simulink model "B2B_HVDC_MMC"  (R2023b)
settings: Solver=ode23t  StartTime=0.0  StopTime=3  FixedStep=Ts_Power  MaxStep=1e-3  MinStep=Ts_Power  RelTol=1e-3
values from neighbouring files (symbols this model uses):
  AC_lim = 1*[1.5 -1.5]    [B2B_HVDC_MMC_Calc.m]
  C_pm = 10.48e-3    (= 0.01048)    [B2B_HVDC_MMC_Calc.m]
  Carm = 1.0*C_pm/n    (= 0.0002096)    [B2B_HVDC_MMC_Calc.m]    (also in HVDC_MMC_param.m = 4.88333333333e-05)
  ccsc_lim = 1*[1.0 -1.0]    [B2B_HVDC_MMC_Calc.m]
  DC_lim = 1*[1.05 -1.05]    [B2B_HVDC_MMC_Calc.m]
  f = 50    [B2B_HVDC_MMC_Calc.m]
  Fn_filter = 1000    [B2B_HVDC_MMC_Calc.m]    (also in HVDC_MMC_param.m)
  Fnom = 50    [HVDC_MMC_param.m]
  HrmOrd = N    (= 2)    [B2B_HVDC_MMC_Calc.m]    (also in HVDC_MMC_param.m)
  I_nom = S_nom/(sqrt(3)*V_grid)    [B2B_HVDC_MMC_Calc.m]
  Ireg_lim_i = 1*[1.5, -1.5]    [B2B_HVDC_MMC_Calc.m]
  Ireg_lim_r = 2*[1.5, -1.5]    [B2B_HVDC_MMC_Calc.m]
  Ki_ACreg_i = 260    [B2B_HVDC_MMC_Calc.m]
  Ki_ccsc = 5    [B2B_HVDC_MMC_Calc.m]
  Ki_DCreg_r = 150    [B2B_HVDC_MMC_Calc.m]
  Ki_Ireg_i = 200    [B2B_HVDC_MMC_Calc.m]
  Ki_Ireg_r = 50    [B2B_HVDC_MMC_Calc.m]
  Kp_ACreg_i = 2    [B2B_HVDC_MMC_Calc.m]
  Kp_ccsc = 1    [B2B_HVDC_MMC_Calc.m]
  Kp_DCreg_r = 8    [B2B_HVDC_MMC_Calc.m]
  Kp_Ireg_i = 2    [B2B_HVDC_MMC_Calc.m]
  Kp_Ireg_r = 0.8    [B2B_HVDC_MMC_Calc.m]
  L1_si = L1_pu*Z_base66/w    [B2B_HVDC_MMC_Calc.m]
  L_arm = L_arm_pu*Z_base66/w    [B2B_HVDC_MMC_Calc.m]
  L_arm_pu = 0.15    [B2B_HVDC_MMC_Calc.m]
  N = 2    [B2B_HVDC_MMC_Calc.m]
  P_nom = 220e6    (= 220000000)    [B2B_HVDC_MMC_Calc.m]
  R1_si = R1_pu*Z_base66    [B2B_HVDC_MMC_Calc.m]
  R_arm = 0.03    [B2B_HVDC_MMC_Calc.m]
  R_arm_pu = R_arm/Z_base66    [B2B_HVDC_MMC_Calc.m]
  R_load = 0.6*40    (= 24)    [B2B_HVDC_MMC_Calc.m]
  R_startup = 17    [B2B_HVDC_MMC_Calc.m]    (also in HVDC_MMC_param.m = 400)
  T_fault = 1.4    [B2B_HVDC_MMC_Calc.m]
  Ts = Ts_Power    (= 5e-05)    [B2B_HVDC_MMC_Calc.m]    (also in HVDC_MMC_param.m)
  Ts_Control = Ts_Power    (= 5e-05)    [B2B_HVDC_MMC_Calc.m]    (also in HVDC_MMC_param.m)
  Ts_DQN = MultTs*Ts_Power    (= 5e-05)    [B2B_HVDC_MMC_Calc.m]    (also in HVDC_MMC_param.m)
  Ts_Power = 1*50e-6    (= 5e-05)    [B2B_HVDC_MMC_Calc.m]    (also in HVDC_MMC_param.m)
  V_ac_ref = 1.035    [B2B_HVDC_MMC_Calc.m]
  V_grid = 66e3    (= 66000)    [B2B_HVDC_MMC_Calc.m]
  Vdc_nom = 135e3    (= 135000)    [B2B_HVDC_MMC_Calc.m]
  Vnom_prim = 333e3    (= 333000)    [HVDC_MMC_param.m]
  Xdcpnz = [zeros(6,1), Xpnz]    [B2B_HVDC_MMC_Calc.m]
  Zeta_filter = 1    [B2B_HVDC_MMC_Calc.m]    (also in HVDC_MMC_param.m)
undefined symbols (not defined in the file or in its folder): DiscIntNeverNeededParam, Pcc, Xdcpnz_c
libraries: DQN_Lib x39, simulink x26, eeTransforms x21, spsCurrentMeasurementLib x16, spsHalfBridgeMMCLib x12, spsSeriesRLCBranchLib x12, B2B_HVDC_MMC_Lib x8, spsSecondOrderFilterLib x8, spsAlphaBetaZerotodq0Lib x6, spsabctoAlphaBetaZeroLib x6, spsThreePhaseVIMeasurementLib x4, spsabctodq0Lib x3
(part 3 of 5)

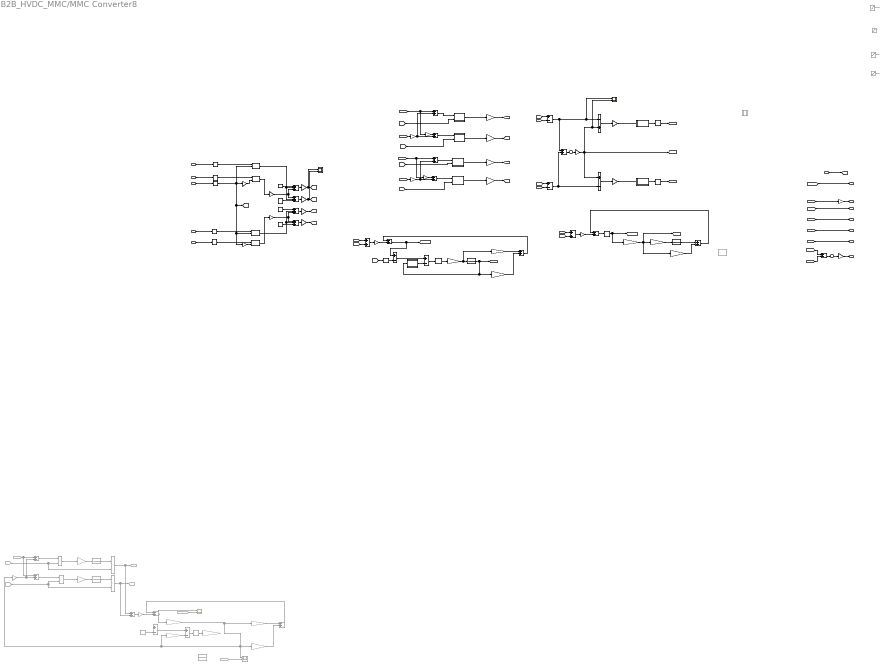
== system B2B_HVDC_MMC/MMC Converter8 ==
  m_dq1_r : Inport
  m_dq2_r : Inport  Port=2
  Vg : Inport  Port=3
  wt : Inport  Port=4
  m_dq1_i : Inport  Port=5
  m_dq2_i : Inport  Port=6
  Add1 : Sum  Inputs=+-
  Add{3,6,38..39,41,44,48,50,73} (9 alike) : Sum
  Add35 : Sum  Commented=on
  Add36 : Sum  Commented=on
  Add37 : Sum  Commented=on  Inputs=-+
  Add4 : Sum  Commented=on
  Add42 : Sum  Inputs=-+
  Add45 : Sum  Inputs=-+
  Add46 : Sum  Inputs=+-
  Add47 : Sum  Inputs=+-
  Add5 : Sum  Commented=on  Inputs=-+
  Constant : Constant  Commented=on  Value=0
  Constant{1..2,74..75} (4 alike) : Constant
  Delay{2..3,8..9} (4 alike) : Delay  DelayLength=1  SampleTime=Ts_Power
  Delay4 : Delay  Commented=on  DelayLength=1  SampleTime=Ts_Power
  Discrete Derivative : simulink/Discrete/Discrete Derivative  Commented=on  gainval=Ts_Power  ICPrevScaledInput=0.0  OutMin=[]  OutMax=[]  OutDataType=fixdt(1, 16)  OutScaling=2^-10  DoSatur=off
  Discrete-Time Integrator : DiscreteIntegrator  IntegratorMethod=Integration: Trapezoidal  SampleTime=Ts_Power  ICPrevOutput=DiscIntNeverNeededParam  ICPrevScaledInput=DiscIntNeverNeededParam
  Discrete-Time Integrator4 : DiscreteIntegrator  Commented=on  IntegratorMethod=Integration: Trapezoidal  SampleTime=Ts_Power  ICPrevOutput=DiscIntNeverNeededParam  ICPrevScaledInput=DiscIntNeverNeededParam
  Discrete-Time Integrator5 : DiscreteIntegrator  Commented=on  IntegratorMethod=Integration: Trapezoidal  SampleTime=Ts_Power  ICPrevOutput=DiscIntNeverNeededParam  ICPrevScaledInput=DiscIntNeverNeededParam
  Discrete-Time Integrator7 : DiscreteIntegrator  IntegratorMethod=Integration: Trapezoidal  SampleTime=Ts_Power  ICPrevOutput=DiscIntNeverNeededParam  ICPrevScaledInput=DiscIntNeverNeededParam
  Discrete-Time Integrator8 : DiscreteIntegrator  Commented=on  IntegratorMethod=Integration: Trapezoidal  SampleTime=Ts_Power  ICPrevOutput=DiscIntNeverNeededParam  ICPrevScaledInput=DiscIntNeverNeededParam
  From108 : From  Commented=on  GotoTag=Id_abc_i
  From51 : From  Commented=on  GotoTag=mn_i
  From56 : From  Commented=on  GotoTag=mp_i
  From72 : From  Commented=on  GotoTag=Ig_abc_i
  From75 : From  Commented=on  GotoTag=Vconv_i
  Gain{1..2,18,23..24} (5 alike) : Gain  Gain=-1
  Gain10 : Gain  Gain=1/6
  Gain12 : Gain  Gain=-2
  Gain13 : Gain  Commented=on  Gain=1/(Carm)
  Gain14 : Gain  Commented=on  Gain=1/(Carm)
  Gain15 : Gain  Commented=on  Gain=0.5
  Gain{3..6} (4 alike) : Gain  Gain=1/(Carm)
  Gain40 : Gain  Commented=on  Gain=-0.5
  Gain41 : Gain  Gain=1/2
  Gain44 : Gain  Gain=0.5
  Gain46 : Gain  Commented=on  Gain=1/R_load
  Gain47 : Gain  Gain=0.5
  Gain49 : Gain  Gain=-0.5
  Gain50 : Gain  Gain=1/R_load
  Gain51 : Gain  Gain=R_arm/2
  Gain52 : Gain  Commented=on  Gain=R_arm/2
  Gain53 : Gain  Commented=on  Gain=L_arm/2
  Gain54 : Gain  Commented=on  Gain=1/L1_si
  Gain55 : Gain  Commented=on  Gain=R1_si+R_load
  Gain56 : Gain  Gain=L_arm/2
  Gain60 : Gain  Gain=-0.5
  Gain61 : Gain  Gain=R_arm/2
  Gain62 : Gain  Gain=L_arm/2
  Gain65 : Gain  Gain=1/L1_si
  Gain9 : Gain  Gain=-2
  Goto56 : Goto  Commented=on  GotoTag=Vp_ic
  Goto57 : Goto  Commented=on  GotoTag=Vn_ic
  I->pu{1..3,5,22,28} (6 alike) : Gain  Gain=1/2  SaturateOnIntegerOverflow=on  OutDataTypeStr=Inherit: Same as input  ParamDataTypeStr=Inherit: Same as input
  Int : MATLAB Function  TreatAsAtomicUnit=on  mask{dt=Ts_Power}
      mask prompts: dt "Time step (s):"
  Int2 : MATLAB Function  TreatAsAtomicUnit=on  mask{dt=Ts_Power}
      mask prompts: dt "Time step (s):"
  Inverse Park Transform{1..4} (4 alike) : eeTransforms/Inverse Park Transform  AxisAlignment=Q-axis  PowerInvariant=off
  MATLAB Function1 : MATLAB Function  TreatAsAtomicUnit=on  mask{dt=Ts_Power}
      mask prompts: dt "Time step (s):"
  MATLAB Function2 : MATLAB Function  TreatAsAtomicUnit=on  mask{dt=Ts_Power}
      mask prompts: dt "Time step (s):"
  MATLAB Function3 : MATLAB Function  TreatAsAtomicUnit=on  mask{dt=Ts_Power}
      mask prompts: dt "Time step (s):"
  MATLAB Function4 : MATLAB Function  TreatAsAtomicUnit=on  mask{dt=Ts_Power}
      mask prompts: dt "Time step (s):"
  Product{1..3,5} (4 alike) : Product  Commented=on
  R_rec1 : Subsystem
  Rate Transition{1..4,10..11} (6 alike) : RateTransition  Integrity=off  OutPortSampleTimeMultiple=MultTs  OutPortSampleTime=Ts_Power
  Saturation3 : Saturate  Commented=on  UpperLimit=inf  LowerLimit=0  ZeroCross=off
  Saturation4 : Saturate  Commented=on  UpperLimit=inf  LowerLimit=0  ZeroCross=off
  Saturation5 : Saturate  Commented=on  UpperLimit=0  LowerLimit=-inf  ZeroCross=off
  Saturation6 : Saturate  Commented=on  UpperLimit=0  LowerLimit=-inf  ZeroCross=off
  Scope : Scope  NumInputPorts=2
  Scope1 : Scope  NumInputPorts=2
  Scope15 : Scope  Commented=on  NumInputPorts=2
  Scope8 : Scope  Commented=on  NumInputPorts=2
  Subsystem2 : Subsystem  Commented=on  mask{Ts_Power=Ts_Power, SW=off}
      mask prompts: Ts_Power "Sample time (s):"; SW "Fancy delay"
  Subtract1 : Sum  Inputs=+-+
  Subtract10 : Sum  Inputs=+-
  Subtract11 : Sum  Inputs=+-
  Subtract2 : Sum  Inputs=+-+
  Subtract3 : Sum  Inputs=+++
  Subtract4 : Sum  Commented=on  Inputs=+-
  Subtract5 : Sum  Inputs=+++
  Subtract8 : Sum  Commented=on  Inputs=+-
  Sum11 : Sum  Inputs=+-  InputSameDT=on  SaturateOnIntegerOverflow=on  OutDataTypeStr=Inherit: Same as first input
  Sum19 : Sum  Inputs=+
  Sum23 : Sum  Inputs=+
  Sum4 : Sum  Inputs=-+  InputSameDT=on  SaturateOnIntegerOverflow=on  OutDataTypeStr=Inherit: Same as first input
  Id_abc_i : Outport  VectorParamsAs1DForOutWhenUnconnected=off
  Ig_abc_i : Outport  Port=2  VectorParamsAs1DForOutWhenUnconnected=off
  Vg_abc_i : Outport  Port=3  VectorParamsAs1DForOutWhenUnconnected=off
  Idc : Outport  Port=4  VectorParamsAs1DForOutWhenUnconnected=off
  Ig_abc_r : Outport  Port=5  VectorParamsAs1DForOutWhenUnconnected=off
  Id_abc_r : Outport  Port=6  VectorParamsAs1DForOutWhenUnconnected=off
  Vdc : Outport  Port=7  VectorParamsAs1DForOutWhenUnconnected=off
  wires:
  Gain9/1 -> Inverse Park Transform2/2
  [mn_r] -> MATLAB Function1/2(y)
  Add6/1 -> MATLAB Function1/1(x)
  Add46/1 -> Scope1/1, Sum4/1, Add73/1  "dVp_M"
  Subtract2/1 -> I->pu22/1
  Constant74/1 -> Subtract2/1
  Inverse Park Transform2/1 -> Gain1/1
  Constant75/1 -> Subtract5/3
  Subtract5/1 -> I->pu28/1
  I->pu28/1 -> Scope/2, [mn_r]
  Inverse Park Transform1/1 -> Subtract5/2, Subtract2/2
  Gain12/1 -> Inverse Park Transform4/2
  wt/1 -> Rate Transition1/1
  Constant2/1 -> Subtract3/3
  Subtract1/1 -> I->pu2/1
  Constant1/1 -> Subtract1/1
  Subtract3/1 -> I->pu3/1
  I->pu2/1 -> [mp_i]
  Inverse Park Transform4/1 -> Gain2/1
  I->pu3/1 -> [mn_i]
  Gain15/1 -> Add4/2, Add5/2
  Discrete-Time Integrator5/1 -> Product2/1  "Vp_M"
  Add5/1 -> Product3/1
  Add4/1 -> Product1/1  "prod"
  Gain14/1 -> Discrete-Time Integrator5/1  "dVp_M"
  Product1/1 -> Gain14/1
  Discrete-Time Integrator4/1 -> Product5/1  "Vn_M"
  Gain13/1 -> Discrete-Time Integrator4/1  "dVn_M"
  Product3/1 -> Gain13/1
  From51/1 -> Product2/2, Product1/2
  From56/1 -> Product3/2, Product5/2
  Vg/1 -> [Vg_r]
  Sum4/1 -> I->pu5/1
  Gain23/1 -> Ig_abc_r/1
  Gain44/1 -> Add6/2, Add3/2
  From75/1 -> Scope8/2
  Constant/1 -> Subtract4/2
  Delay4/1 -> Gain54/1
  Gain55/1 -> Subtract8/2
  Subtract8/1 -> Delay4/1
  Gain53/1 -> Add36/1  "dVp_M"
  Gain52/1 -> Add36/2  "dVp_M"
  Add37/1 -> Scope8/1, Gain46/1  "prod"
  Subtract4/1 -> Subtract8/1
  Product2/1 -> Add35/1, Goto56/1
  Gain46/1 -> Scope15/1, Gain55/1, Gain15/1, Gain52/1, Gain53/1  "Igd"
  Product5/1 -> Add35/2, Goto57/1
  From72/1 -> Scope15/2
  Add36/1 -> Add37/1  "prod"
  Add35/1 -> Gain40/1
  Gain40/1 -> Add37/2  "Vce_i"
  From108/1 -> Add5/1, Add4/1
  Gain47/1 -> Add38/2, Add39/2
  [mp_i] -> MATLAB Function4/2(y)
  Add38/1 -> MATLAB Function3/1(x)  "prod"
  Add39/1 -> MATLAB Function4/1(x)
  [mn_i] -> MATLAB Function3/2(y)
  Add41/1 -> Add42/1  "prod"
  Gain51/1 -> Add41/2  "dVp_M"
  Add50/1 -> Gain49/1
  Gain49/1 -> Add42/2  "Vce_i"
  Subtract10/1 -> Subtract11/1
  Gain61/1 -> Add44/2  "dVp_M"
  Add44/1 -> Add45/1  "prod"
  Gain60/1 -> Add45/2  "Vce_r"
  Gain62/1 -> Add44/1  "dVp_M"
  R_rec1/1(Out) -> Subtract11/2
  Gain65/1 -> Discrete-Time Integrator/1, Gain62/1
  Add48/1 -> Gain60/1
  [Ig_abc_ic] -> Gain47/1
  [Id_abc_ic] -> Gain24/1, Add38/1
  [Vp_rc] -> Add46/1
  [Vn_rc] -> Add46/2
  [Vp_ic] -> Add47/1
  [Vn_ic] -> Add47/2
  [Ig_abc_rc] -> Gain44/1
  [Id_abc_rc] -> Add3/1, Gain18/1
  [Vp_rc] -> Add48/1
  [Vn_rc] -> Add48/2
  [Vp_ic] -> Add50/1
  [Vn_ic] -> Add50/2
  Add47/1 -> Sum11/2, Add73/2  "dVp_M"
  [Ig_abc_rc] -> Gain23/1
  [Id_abc_rc] -> Id_abc_r/1
  [Ig_abc_ic] -> Ig_abc_i/1
  [Id_abc_ic] -> Id_abc_i/1
  [Id_abc_rc] -> Add1/2
  Gain56/1 -> Discrete-Time Integrator7/1  "dVp_M"
  Discrete-Time Integrator7/1 -> Add41/1
  [Id_abc_ic] -> Add1/1
  Add1/1 -> Sum23/1
  Gain41/1 -> Idc/1  "Vce_r"
  Discrete-Time Integrator/1 -> [Ig_abc_rc], R_rec1/1(In), Gain61/1  "Igd"
  Add45/1 -> [Vconv_rc], Subtract10/1  "prod"
  Gain50/1 -> Gain51/1, [Ig_abc_ic], Gain56/1  "Igd"
  Add42/1 -> Delay8/1  "prod"
  [Vconv_ic] -> Vg_abc_i/1
  [V_dc_c] -> Vdc/1
  Subtract11/1 -> Delay9/1
  Gain1/1 -> Subtract5/1, Subtract2/3
  Inverse Park Transform3/1 -> Subtract1/2, Subtract3/2
  Gain2/1 -> Subtract3/1, Subtract1/3
  Gain10/1 -> Sum11/1, Scope1/2, Sum4/2, [V_dc_c]  "Vce_r"
  m_dq2_r/1 -> Rate Transition11/1
  m_dq1_r/1 -> Rate Transition10/1
  m_dq1_i/1 -> Rate Transition2/1
  m_dq2_i/1 -> Rate Transition3/1
  Gain18/1 -> Add6/1
  Gain24/1 -> Add39/1
  Saturation4/1 -> ?
  Saturation3/1 -> ?
  Saturation6/1 -> ?
  Add73/1 -> Sum19/1
  Sum19/1 -> Gain10/1
  Int/1(z) -> Delay2/1
  Sum11/1 -> I->pu1/1
  Int2/1(z) -> Delay3/1
  MATLAB Function3/1(z) -> Gain5/1
  MATLAB Function4/1(z) -> Gain6/1
  Delay2/1 -> [Id_abc_rc]
  Delay3/1 -> [Id_abc_ic]
  Delay9/1 -> Gain65/1
  Delay8/1 -> Gain50/1, [Vconv_ic]
  I->pu5/1 -> Int/1(x)
  I->pu1/1 -> Int2/1(x)
  Rate Transition10/1 -> Inverse Park Transform1/1
  Rate Transition11/1 -> Inverse Park Transform2/1
  Rate Transition1/1 -> [wt], Inverse Park Transform3/2, Gain12/1, Inverse Park Transform1/2, Gain9/1
  Rate Transition2/1 -> Inverse Park Transform3/1
  Rate Transition3/1 -> Inverse Park Transform4/1
  [Vg_r] -> Rate Transition4/1
  Rate Transition4/1 -> Subtract10/2
  Sum23/1 -> Gain41/1
  I->pu22/1 -> Scope/1, [mp_r]
  Add3/1 -> MATLAB Function2/1(x)  "prod"
  [mp_r] -> MATLAB Function2/2(y)
  MATLAB Function2/1(z) -> Gain3/1  "dVp_M"
  Gain3/1 -> [Vp_rc]  "dVp_M"
  MATLAB Function1/1(z) -> Gain4/1  "dVp_M"
  Gain4/1 -> [Vn_rc]  "dVp_M"
  Gain5/1 -> [Vp_ic]  "dVp_M"
  Gain6/1 -> [Vn_ic]  "dVp_M"

== system B2B_HVDC_MMC/Dq0 Control11/Subsystem1 ==
  V_dc_meas : Inport
  Ig_dq1+ : Inport  Port=2
  Vg_dq1+ : Inport  Port=3
  Id_dq2- : Inport  Port=4
  AC Voltage Controller : Subsystem
  Circulating current suppression : Subsystem  VariantControl=Variant1
  Constant1 : Constant  Value=1/(Vdc_nom/2*sqrt(3)/sqrt(2)/V_grid)
  Constant2 : Constant  Value=Vdc_nom
  Constant6 : Constant  Value=V_grid
  DC voltage control - Outer loop : Subsystem
  Gain5 : Gain  Gain=(V_grid)
  Inncer current loop - Positive and Negative Sequence Control : Subsystem
  Interpreted MATLAB Function : MATLABFcn  MATLABFcn=sqrt(u(1)^2+u(2)^2)
  Step : Step  Time=(T_fault+0.15)  Before=[DC_lim(1) DC_lim(2)]  After=[DC_lim(1) DC_lim(2)]  SampleTime=0
  m_dq1 : Outport
  m_dq2 : Outport  Port=2
  wires:
  Interpreted MATLAB Function/1 -> AC Voltage Controller/3(V_ac)
  Vg_dq1+/1 -> Gain5/1, Inncer current loop - Positive and Negative Sequence Control/4(Vdq+)
  [T_circ_r] -> Circulating current suppression/Enable
  [T_iq_reg_r] -> AC Voltage Controller/Enable, AC Voltage Controller/1("Enable ")
  Constant2/1 -> DC voltage control - Outer loop/2(V_dc_ref)
  AC Voltage Controller/1(Iq_ref) -> Inncer current loop - Positive and Negative Sequence Control/2(iq_pos_ref)
  DC voltage control - Outer loop/1(Id_ref) -> Inncer current loop - Positive and Negative Sequence Control/1(id_pos_ref)
  [T_DC_Reg] -> DC voltage control - Outer loop/3(Enable)
  Step/1 -> DC voltage control - Outer loop/4(DC_limit)
  Constant6/1 -> AC Voltage Controller/2(V_ac_ref)
  Gain5/1 -> Interpreted MATLAB Function/1
  Constant1/1 -> Inncer current loop - Positive and Negative Sequence Control/5(Vdc_pu)
  V_dc_meas/1 -> DC voltage control - Outer loop/1(V_dc_meas)
  Ig_dq1+/1 -> Inncer current loop - Positive and Negative Sequence Control/3(Idq+)
  Circulating current suppression/1(m_dq2) -> m_dq2/1
  Inncer current loop - Positive and Negative Sequence Control/1(m_dq1) -> m_dq1/1
  Id_dq2-/1 -> Circulating current suppression/1(I_arm)

== system B2B_HVDC_MMC/Dq0 Control8/Subsystem ==
  vdq+ : Inport
  Idq+ : Inport  Port=2
  Id_dq2- : Inport  Port=3
  Add : Sum  Inputs=1
  Circulating current suppression : Subsystem  VariantControl=Variant1
  Constant18 : Constant  Value=V_ac_ref
  Constant2 : Constant  Value=1/(Vdc_nom/2*sqrt(3)/sqrt(2)/V_grid)
  Demux5 : Demux  Outputs=2
  Discrete Mean value4 : powerlib_extras/Discrete Measurements/Discrete  Mean value  Freq=f  Vinit=0  Ts=Ts_Power
  Discrete Mean value5 : powerlib_extras/Discrete Measurements/Discrete  Mean value  Freq=f  Vinit=0  Ts=Ts_Power
  Inncer current loop - Positive and Negative Sequence Control : Subsystem
  Mux6 : Mux  Inputs=2
  Outer loop - AC RMS controller1 : Subsystem
  Product1 : Product  RndMeth=Zero
  Product2 : Product  RndMeth=Zero
  Reactive power Set-point : Subsystem
  Second-Order Filter1 : spsSecondOrderFilterLib/Second-Order Filter  FilterType=Lowpass  Fo=Fn_filter  Zeta=Zeta_filter  Ts=Ts_Control  Initialize=off  Vac_Init="[0,  0,  60]"  Vdc_Init=0  PlotResponse=off  FreqRange=[0, 500, 1]
  Second-Order Filter2 : spsSecondOrderFilterLib/Second-Order Filter  FilterType=Lowpass  Fo=Fn_filter  Zeta=Zeta_filter  Ts=Ts_Control  Initialize=off  Vac_Init="[0,  0,  60]"  Vdc_Init=0  PlotResponse=off  FreqRange=[0, 500, 1]
  Second-Order Filter5 : spsSecondOrderFilterLib/Second-Order Filter  FilterType=Lowpass  Fo=Fn_filter  Zeta=Zeta_filter  Ts=Ts_Control  Initialize=off  Vac_Init="[0,  0,  60]"  Vdc_Init=0  PlotResponse=off  FreqRange=[0, 500, 1]
  Selector4 : Selector  InputPortWidth=2  IndexOptions=Index vector (dialog)  Indices=[2 1]  OutputSizes=1
  Subtract : Sum  Inputs=+-
  m_dq1 : Outport
  m_dq2 : Outport  Port=2
  wires:
  [T_AC_Reg] -> Outer loop - AC RMS controller1/3(Enable)
  Reactive power Set-point/1(Iq_ref) -> Inncer current loop - Positive and Negative Sequence Control/2(iq_pos_ref)
  Mux6/1 -> Reactive power Set-point/2(Q_ref)
  Constant2/1 -> Inncer current loop - Positive and Negative Sequence Control/5(Vdc_pu)
  [T_iq_reg_i] -> Reactive power Set-point/Enable, Reactive power Set-point/1(T_Qreg_on)
  Constant18/1 -> Outer loop - AC RMS controller1/1(Vac_ref)
  [T_circ_i] -> Circulating current suppression/Enable
  Outer loop - AC RMS controller1/1(Id_ref) -> Inncer current loop - Positive and Negative Sequence Control/1(id_pos_ref)
  Inncer current loop - Positive and Negative Sequence Control/1(m_dq1) -> m_dq1/1
  Second-Order Filter2/1 -> Circulating current suppression/1(Id_dq2-)
  Circulating current suppression/1(m_dq2) -> m_dq2/1
  Add/1 -> Discrete Mean value5/1  "P_i"
  Discrete Mean value5/1 -> Mux6/1
  vdq+/1 -> Second-Order Filter5/1
  Discrete Mean value4/1 -> Mux6/2
  Product2/1 -> Demux5/1
  Subtract/1 -> Discrete Mean value4/1
  Selector4/1 -> Product2/1
  Product1/1 -> Add/1
  Demux5/1 -> Subtract/1
  Idq+/1 -> Second-Order Filter1/1
  Demux5/2 -> Subtract/2
  Second-Order Filter5/1 -> Outer loop - AC RMS controller1/2(vdq+), Inncer current loop - Positive and Negative Sequence Control/4(Vdq+), Reactive power Set-point/3(Vdq+), Selector4/1, Product1/1
  Second-Order Filter1/1 -> Product2/2, Product1/2, Inncer current loop - Positive and Negative Sequence Control/3(Idq+)
  Id_dq2-/1 -> Second-Order Filter2/1

== system B2B_HVDC_MMC/MMC Converter2/R_rec1 ==
  In : Inport
  Gain29 : Gain  Gain=R1_si
  Gain47 : Gain  Gain=R1_si+R_startup
  Switch3 : Switch  Criteria=u2 > Threshold  SaturateOnIntegerOverflow=off  InputSameDT=off
  Out : Outport
  wires:
  Gain47/1 -> Switch3/3
  In/1 -> Gain47/1, Gain29/1
  Gain29/1 -> Switch3/1
  [T_startup] -> Switch3/2
  Switch3/1 -> Out/1

== system B2B_HVDC_MMC/MMC Converter2/Subsystem2 ==
  In1 : Inport
  Constant : Constant  Value=SW
  Gain38 : Gain  Gain=2
  Sum2 : Sum  Inputs=+-  InputSameDT=on  SaturateOnIntegerOverflow=on  OutDataTypeStr=Inherit: Same as first input
  Switch : Switch  Criteria=u2 > Threshold  Threshold=0.5  SaturateOnIntegerOverflow=off  InputSameDT=off
  Unit Delay3 : UnitDelay  SampleTime=Ts_Power  HasFrameUpgradeWarning=on
  Unit Delay4 : UnitDelay  SampleTime=Ts_Power  HasFrameUpgradeWarning=on
  Out1 : Outport
  wires:
  Gain38/1 -> Sum2/1
  Unit Delay4/1 -> Switch/3, Unit Delay3/1, Gain38/1
  In1/1 -> Unit Delay4/1
  Unit Delay3/1 -> Sum2/2
  Sum2/1 -> Switch/1
  Constant/1 -> Switch/2
  Switch/1 -> Out1/1

== system B2B_HVDC_MMC/MMC Converter3/Subsystem5 ==
  Brk1 : spsThreePhaseBreakerLib/Three-Phase Breaker  InitialState=open  SwitchA=on  SwitchB=on  SwitchC=on  SwitchTimes=[30/60]*10000  External=on  BreakerResistance=0.01  SnubberResistance=1e6  SnubberCapacitance=inf  Measurements=None  mask(Three-Phase Breaker){}
  R_startup : spsThreePhaseSeriesRLCBranchLib/Three-Phase Series RLC Branch  LConnTagsString=A|B|C  RConnTagsString=A|B|C  BranchType=R  Resistance=R_startup  Inductance=Vnom_prim^2 / Pcc / (2*pi*Fnom)  Capacitance=1e-6  Measurements=None
  Scope : Scope  Commented=on
  Voltage Measurement1 : spsVoltageMeasurementLib/Voltage Measurement  Commented=on  PhasorSimulation=off  OutputType=Complex  PSBequivalent=0
  a : PMIOPort  Side=Left
  A : PMIOPort  Port=2  Side=Right
  b : PMIOPort  Port=3  Side=Left
  B : PMIOPort  Port=4  Side=Right
  c : PMIOPort  Port=5  Side=Left
  C : PMIOPort  Port=6  Side=Right
  wires:
  Voltage Measurement1/1 -> Scope/1
  [T_startup] -> Brk1/1
  connections:
  R_startup/RConn1 -- A/RConn1 -- Brk1/RConn1
  R_startup/LConn1 -- a/RConn1 -- Brk1/LConn1
  R_startup/RConn2 -- B/RConn1 -- Brk1/RConn2
  Voltage Measurement1/LConn1 -- c/RConn1 -- Brk1/LConn3 -- R_startup/LConn3
  R_startup/LConn2 -- b/RConn1 -- Brk1/LConn2
  R_startup/RConn3 -- C/RConn1 -- Voltage Measurement1/LConn2 -- Brk1/RConn3

== system B2B_HVDC_MMC/MMC Converter3/Voltage source ==
  In1 : Inport
  Controlled Voltage Source : spsControlledVoltageSourceLib/Controlled Voltage Source  Initialize=on  Source_Type=AC  Amplitude=0  Phase=0  Frequency=f  Measurements=None
  Controlled Voltage Source6 : spsControlledVoltageSourceLib/Controlled Voltage Source  Initialize=on  Source_Type=AC  Amplitude=0  Phase=0  Frequency=0  Measurements=None
  Controlled Voltage Source7 : spsControlledVoltageSourceLib/Controlled Voltage Source  Initialize=on  Source_Type=AC  Amplitude=0  Phase=0  Frequency=0  Measurements=None
  Demux9 : Demux  Outputs=3
  Ground : spsGroundLib/Ground  LConnTagsString=a
  a : PMIOPort  Side=Right
  b : PMIOPort  Port=2  Side=Right
  c : PMIOPort  Port=3  Side=Right
  wires:
  In1/1 -> Demux9/1
  Demux9/1 -> Controlled Voltage Source/1
  Demux9/2 -> Controlled Voltage Source6/1
  Demux9/3 -> Controlled Voltage Source7/1
  connections:
  Ground/LConn1 -- Controlled Voltage Source6/LConn1 -- Controlled Voltage Source/LConn1 -- Controlled Voltage Source7/LConn1
  Controlled Voltage Source7/RConn1 -- c/RConn1
  Controlled Voltage Source6/RConn1 -- b/RConn1
  Controlled Voltage Source/RConn1 -- a/RConn1

== system B2B_HVDC_MMC/MMC Converter4/R_rec2 ==
  In : Inport
  Product : Product
  Step : Step  Time=0.4  Before=R1_si+R_startup  After=R1_si  SampleTime=0
  Out : Outport
  wires:
  Product/1 -> Out/1
  Step/1 -> Product/2
  In/1 -> Product/1

== system B2B_HVDC_MMC/MMC Converter4/Subsystem1 ==
  "{X_DQN}" : Inport
  Demux28 : Demux  Outputs=[Hi+1,Hi+1,Hi+1,Hi+1,Hi+1,Hi+1]
  Mux : Mux  Inputs=[Ho+1,Ho+1,Ho+1,Ho+1,Ho+1,Ho+1]
  Selector{,1..5} (6 alike) : Selector  InputPortWidth=Hi+1  IndexOptions=Index vector (dialog)  Indices=[1:Ho+1]  OutputSizes=1
  "{Y_DQN}" : Outport
  wires:
  Selector5/1 -> Mux/6
  Selector2/1 -> Mux/3
  Demux28/2 -> Selector1/1
  Demux28/1 -> Selector/1
  Demux28/3 -> Selector2/1
  Selector/1 -> Mux/1
  Demux28/4 -> Selector3/1
  Selector1/1 -> Mux/2
  Selector3/1 -> Mux/4
  "{X_DQN}"/1 -> Demux28/1
  Selector4/1 -> Mux/5
  Demux28/5 -> Selector4/1
  Demux28/6 -> Selector5/1
  Mux/1 -> "{Y_DQN}"/1

== system B2B_HVDC_MMC/MMC Converter4/Subsystem2 ==
  "{X_DQN}" : Inport
  Demux28 : Demux  Outputs=[Hi+1,Hi+1,Hi+1,Hi+1,Hi+1,Hi+1]
  Mux : Mux  Inputs=[Ho+1,Ho+1,Ho+1,Ho+1,Ho+1,Ho+1]
  Selector{,1..5} (6 alike) : Selector  InputPortWidth=Hi+1  IndexOptions=Index vector (dialog)  Indices=[1:Ho+1]  OutputSizes=1
  "{Y_DQN}" : Outport
  wires:
  Selector5/1 -> Mux/6
  Selector2/1 -> Mux/3
  Demux28/2 -> Selector1/1
  Demux28/1 -> Selector/1
  Demux28/3 -> Selector2/1
  Selector/1 -> Mux/1
  Demux28/4 -> Selector3/1
  Selector1/1 -> Mux/2
  Selector3/1 -> Mux/4
  "{X_DQN}"/1 -> Demux28/1
  Selector4/1 -> Mux/5
  Demux28/5 -> Selector4/1
  Demux28/6 -> Selector5/1
  Mux/1 -> "{Y_DQN}"/1

== system B2B_HVDC_MMC/MMC Converter4/Subsystem3 ==
  "{X_DQN}" : Inport
  Demux28 : Demux  Outputs=[Hi+1,Hi+1,Hi+1,Hi+1,Hi+1,Hi+1]
  Mux : Mux  Inputs=[Ho+1,Ho+1,Ho+1,Ho+1,Ho+1,Ho+1]
  Selector{,1..5} (6 alike) : Selector  InputPortWidth=Hi+1  IndexOptions=Index vector (dialog)  Indices=[1:Ho+1]  OutputSizes=1
  "{Y_DQN}" : Outport
  wires:
  Selector5/1 -> Mux/6
  Selector2/1 -> Mux/3
  Demux28/2 -> Selector1/1
  Demux28/1 -> Selector/1
  Demux28/3 -> Selector2/1
  Selector/1 -> Mux/1
  Demux28/4 -> Selector3/1
  Selector1/1 -> Mux/2
  Selector3/1 -> Mux/4
  "{X_DQN}"/1 -> Demux28/1
  Selector4/1 -> Mux/5
  Demux28/5 -> Selector4/1
  Demux28/6 -> Selector5/1
  Mux/1 -> "{Y_DQN}"/1

== system B2B_HVDC_MMC/MMC Converter4/Subsystem4 ==
  "{X_DQN}" : Inport
  Demux28 : Demux  Outputs=[Hi+1,Hi+1,Hi+1,Hi+1,Hi+1,Hi+1]
  Mux : Mux  Inputs=[Ho+1,Ho+1,Ho+1,Ho+1,Ho+1,Ho+1]
  Selector{,1..5} (6 alike) : Selector  InputPortWidth=Hi+1  IndexOptions=Index vector (dialog)  Indices=[1:Ho+1]  OutputSizes=1
  "{Y_DQN}" : Outport
  wires:
  Selector5/1 -> Mux/6
  Selector2/1 -> Mux/3
  Demux28/2 -> Selector1/1
  Demux28/1 -> Selector/1
  Demux28/3 -> Selector2/1
  Selector/1 -> Mux/1
  Demux28/4 -> Selector3/1
  Selector1/1 -> Mux/2
  Selector3/1 -> Mux/4
  "{X_DQN}"/1 -> Demux28/1
  Selector4/1 -> Mux/5
  Demux28/5 -> Selector4/1
  Demux28/6 -> Selector5/1
  Mux/1 -> "{Y_DQN}"/1

== system B2B_HVDC_MMC/MMC Converter4/Subsystem5 ==
  "{X_DQN}" : Inport
  Demux28 : Demux  Outputs=[Hi+1,Hi+1,Hi+1,Hi+1,Hi+1,Hi+1]
  Mux : Mux  Inputs=[Ho+1,Ho+1,Ho+1,Ho+1,Ho+1,Ho+1]
  Selector{,1..5} (6 alike) : Selector  InputPortWidth=Hi+1  IndexOptions=Index vector (dialog)  Indices=[1:Ho+1]  OutputSizes=1
  "{Y_DQN}" : Outport
  wires:
  Selector5/1 -> Mux/6
  Selector2/1 -> Mux/3
  Demux28/2 -> Selector1/1
  Demux28/1 -> Selector/1
  Demux28/3 -> Selector2/1
  Selector/1 -> Mux/1
  Demux28/4 -> Selector3/1
  Selector1/1 -> Mux/2
  Selector3/1 -> Mux/4
  "{X_DQN}"/1 -> Demux28/1
  Selector4/1 -> Mux/5
  Demux28/5 -> Selector4/1
  Demux28/6 -> Selector5/1
  Mux/1 -> "{Y_DQN}"/1

== system B2B_HVDC_MMC/MMC Converter4/Subsystem6 ==
  "{X_DQN}" : Inport
  Demux28 : Demux  Outputs=[Hi+1,Hi+1,Hi+1,Hi+1,Hi+1,Hi+1]
  Mux : Mux  Inputs=[Ho+1,Ho+1,Ho+1,Ho+1,Ho+1,Ho+1]
  Selector{,1..5} (6 alike) : Selector  InputPortWidth=Hi+1  IndexOptions=Index vector (dialog)  Indices=[1:Ho+1]  OutputSizes=1
  "{Y_DQN}" : Outport
  wires:
  Selector5/1 -> Mux/6
  Selector2/1 -> Mux/3
  Demux28/2 -> Selector1/1
  Demux28/1 -> Selector/1
  Demux28/3 -> Selector2/1
  Selector/1 -> Mux/1
  Demux28/4 -> Selector3/1
  Selector1/1 -> Mux/2
  Selector3/1 -> Mux/4
  "{X_DQN}"/1 -> Demux28/1
  Selector4/1 -> Mux/5
  Demux28/5 -> Selector4/1
  Demux28/6 -> Selector5/1
  Mux/1 -> "{Y_DQN}"/1

== system B2B_HVDC_MMC/MMC Converter4/Subsystem7 ==
  "{X_DQN}" : Inport
  Demux28 : Demux  Outputs=[Hi+1,Hi+1,Hi+1,Hi+1,Hi+1,Hi+1]
  Mux : Mux  Inputs=[Ho+1,Ho+1,Ho+1,Ho+1,Ho+1,Ho+1]
  Selector{,1..5} (6 alike) : Selector  InputPortWidth=Hi+1  IndexOptions=Index vector (dialog)  Indices=[1:Ho+1]  OutputSizes=1
  "{Y_DQN}" : Outport
  wires:
  Selector5/1 -> Mux/6
  Selector2/1 -> Mux/3
  Demux28/2 -> Selector1/1
  Demux28/1 -> Selector/1
  Demux28/3 -> Selector2/1
  Selector/1 -> Mux/1
  Demux28/4 -> Selector3/1
  Selector1/1 -> Mux/2
  Selector3/1 -> Mux/4
  "{X_DQN}"/1 -> Demux28/1
  Selector4/1 -> Mux/5
  Demux28/5 -> Selector4/1
  Demux28/6 -> Selector5/1
  Mux/1 -> "{Y_DQN}"/1

== system B2B_HVDC_MMC/MMC Converter4/Subsystem8 ==
  "{X_DQN}" : Inport
  Demux28 : Demux  Outputs=[Hi+1,Hi+1,Hi+1,Hi+1,Hi+1,Hi+1]
  Mux : Mux  Inputs=[Ho+1,Ho+1,Ho+1,Ho+1,Ho+1,Ho+1]
  Selector{,1..5} (6 alike) : Selector  InputPortWidth=Hi+1  IndexOptions=Index vector (dialog)  Indices=[1:Ho+1]  OutputSizes=1
  "{Y_DQN}" : Outport
  wires:
  Selector5/1 -> Mux/6
  Selector2/1 -> Mux/3
  Demux28/2 -> Selector1/1
  Demux28/1 -> Selector/1
  Demux28/3 -> Selector2/1
  Selector/1 -> Mux/1
  Demux28/4 -> Selector3/1
  Selector1/1 -> Mux/2
  Selector3/1 -> Mux/4
  "{X_DQN}"/1 -> Demux28/1
  Selector4/1 -> Mux/5
  Demux28/5 -> Selector4/1
  Demux28/6 -> Selector5/1
  Mux/1 -> "{Y_DQN}"/1

== system B2B_HVDC_MMC/MMC Converter8/R_rec1 ==
  In : Inport
  Gain29 : Gain  Gain=R1_si
  Gain47 : Gain  Gain=R1_si+R_startup
  Switch3 : Switch  Criteria=u2 > Threshold  SaturateOnIntegerOverflow=off  InputSameDT=off
  Out : Outport
  wires:
  Gain47/1 -> Switch3/3
  In/1 -> Gain47/1, Gain29/1
  Gain29/1 -> Switch3/1
  [T_startup] -> Switch3/2
  Switch3/1 -> Out/1

== system B2B_HVDC_MMC/MMC Converter8/Subsystem2 ==
  In1 : Inport
  Constant : Constant  Value=SW
  Gain38 : Gain  Gain=2
  Sum2 : Sum  Inputs=+-  InputSameDT=on  SaturateOnIntegerOverflow=on  OutDataTypeStr=Inherit: Same as first input
  Switch : Switch  Criteria=u2 > Threshold  Threshold=0.5  SaturateOnIntegerOverflow=off  InputSameDT=off
  Unit Delay3 : UnitDelay  SampleTime=Ts_Power  HasFrameUpgradeWarning=on
  Unit Delay4 : UnitDelay  SampleTime=Ts_Power  HasFrameUpgradeWarning=on
  Out1 : Outport
  wires:
  Gain38/1 -> Sum2/1
  Unit Delay4/1 -> Switch/3, Unit Delay3/1, Gain38/1
  In1/1 -> Unit Delay4/1
  Unit Delay3/1 -> Sum2/2
  Sum2/1 -> Switch/1
  Constant/1 -> Switch/2
  Switch/1 -> Out1/1

== system B2B_HVDC_MMC/Dq0 Control11/Subsystem1/AC Voltage Controller ==
  "Enable " : Inport
  V_ac_ref : Inport  Port=2
  V_ac : Inport  Port=3
  Enable : EnablePort
  Gain1 : Gain  Gain=1/V_grid
  Gain2 : Gain  Gain=-1
  PID Controller : simulink/Continuous/PID Controller  Controller=PI  Form=Parallel  TimeDomain=Continuous-time  UseExternalTs=off  SampleTime=-1  IntegratorMethod=Forward Euler  ControllerParametersSource=internal  P=2  I=40  D=0  UseFilter=on  N=100  TunerSelectOption=Transfer Function Based (PID Tuner App)  InitialConditionSource=internal  InitialConditionForIntegrator=0  InitialConditionForFilter=0  DifferentiatorICPrevScaledInput=0  ExternalReset=none  TrackingMode=off  Kt=1  LimitOutput=off  UpperSaturationLimit=inf  LowerSaturationLimit=-inf  LinearizeAsGain=on  AntiWindupMode=none  Kb=1  POutMin=[]  POutMax=[]  IOutMin=[]  IOutMax=[]  DOutMin=[]  DOutMax=[]  NOutMin=[]  NOutMax=[]  SumOutMin=[]  SumOutMax=[]  SaturationOutMin=[]  SaturationOutMax=[]  PParamMin=[]  PParamMax=[]  IParamMin=[]  IParamMax=[]  DParamMin=[]  DParamMax=[]  NParamMin=[]  NParamMax=[]  KbParamMin=[]  KbParamMax=[]  KtParamMin=[]  KtParamMax=[]  KbOutMin=[]  KbOutMax=[]  KtOutMin=[]  KtOutMax=[]  IntegratorOutMin=[]  IntegratorOutMax=[]  FilterOutMin=[]  FilterOutMax=[]  SumI1OutMin=[]  SumI1OutMax=[]  SumI2OutMin=[]  SumI2OutMax=[]  SumI3OutMin=[]  SumI3OutMax=[]  SumI4OutMin=[]  SumI4OutMax=[]  SumDOutMin=[]  SumDOutMax=[]  DifferentiatorOutMin=[]  DifferentiatorOutMax=[]  FilterDiffOutCoefMin=[]  FilterDiffOutCoefMax=[]  ReciprocalOutMin=[]  ReciprocalOutMax=[]  SumDenOutMin=[]  SumDenOutMax=[]  SumNumOutMin=[]  SumNumOutMax=[]  DivideOutMin=[]  DivideOutMax=[]  UdiffTsProdOutMin=[]  UdiffTsProdOutMax=[]  NTsProdOutMin=[]  NTsProdOutMax=[]  UintegralTsProdOutMin=[]  UintegralTsProdOutMax=[]  UngainTsProdOutMin=[]  UngainTsProdOutMax=[]  IntegratorContinuousStateAttributes=''  IntegratorStateMustResolveToSignalObject=off  IntegratorRTWStateStorageClass=Auto  FilterContinuousStateAttributes=''  FilterStateMustResolveToSignalObject=off  FilterRTWStateStorageClass=Auto  ParallelPVariant=InternalParameters  IdealPVariant=Disabled  IVariant=InternalParameters  DVariant=Disabled  IntegratorVariant=Continuous  SatVariant=Disabled  AWVariant=Passthrough  PCopyVariant=Disabled  TRVariant=Disabled  FdbkBlocksVariant=Forward  IdealPFdbkVariant=Disabled  SatFdbkVariant=Disabled  DerivativeFilterVariant=Disabled  NVariant=Disabled  NCopyVariant=Disabled_SignalSpec  FilterICVariant=Disabled  IntegratorICVariant=InternalICs  ExternalResetVariant=Disabled  TRSumVariant=Passthrough  SumFdbkVariant=Disabled  SumVariant=Sum_PI  TsampFilterVariant=InternalTs  TsampNgainVariant=Passthrough  TsampIntegralVariant=Passthrough
  Rate Transition14 : RateTransition  OutPortSampleTime=Ts_Control
  Saturation : Saturate  UpperLimit=1  LowerLimit=-1
  Sum : Sum  Inputs=|+-
  Switch : Switch  Criteria=u2 > Threshold  SaturateOnIntegerOverflow=off  InputSameDT=off
  Unit Delay : UnitDelay  SampleTime=Ts_Power  HasFrameUpgradeWarning=on
  Iq_ref : Outport  VectorParamsAs1DForOutWhenUnconnected=off
  wires:
  Gain2/1 -> Iq_ref/1, [iq_ref_r]
  Saturation/1 -> Gain2/1
  Sum/1 -> Gain1/1
  Switch/1 -> Sum/1
  V_ac_ref/1 -> Switch/1
  Unit Delay/1 -> Rate Transition14/1
  "Enable "/1 -> Switch/2
  V_ac/1 -> Unit Delay/1
  PID Controller/1 -> Saturation/1
  Rate Transition14/1 -> ?
  Gain1/1 -> PID Controller/1
  ? -> Switch/3, Sum/2

== system B2B_HVDC_MMC/Dq0 Control11/Subsystem1/Circulating current suppression ==
  I_arm : Inport
  Enable1 : EnablePort
  Constant1 : Constant  Value=0
  Constant2 : Constant  Value=0
  Constant4 : Constant  Value=0
  Demux : Demux  Outputs=2
  Discrete PID Controller : simulink/Continuous/PID Controller  Controller=PI  Form=Parallel  TimeDomain=Discrete-time  UseExternalTs=off  SampleTime=Ts_Power  IntegratorMethod=Forward Euler  ControllerParametersSource=internal  P=Kp_ccsc  I=Ki_ccsc  D=0  UseFilter=on  N=100  TunerSelectOption=Transfer Function Based (PID Tuner App)  InitialConditionSource=internal  InitialConditionForIntegrator=0  InitialConditionForFilter=0  DifferentiatorICPrevScaledInput=0  ExternalReset=none  TrackingMode=off  Kt=1  LimitOutput=off  UpperSaturationLimit=inf  LowerSaturationLimit=-inf  LinearizeAsGain=off  AntiWindupMode=none  Kb=1  POutMin=[]  POutMax=[]  IOutMin=[]  IOutMax=[]  DOutMin=[]  DOutMax=[]  NOutMin=[]  NOutMax=[]  SumOutMin=[]  SumOutMax=[]  SaturationOutMin=[]  SaturationOutMax=[]  PParamMin=[]  PParamMax=[]  IParamMin=[]  IParamMax=[]  DParamMin=[]  DParamMax=[]  NParamMin=[]  NParamMax=[]  KbParamMin=[]  KbParamMax=[]  KtParamMin=[]  KtParamMax=[]  KbOutMin=[]  KbOutMax=[]  KtOutMin=[]  KtOutMax=[]  IntegratorOutMin=[]  IntegratorOutMax=[]  FilterOutMin=[]  FilterOutMax=[]  SumI1OutMin=[]  SumI1OutMax=[]  SumI2OutMin=[]  SumI2OutMax=[]  SumI3OutMin=[]  SumI3OutMax=[]  SumI4OutMin=[]  SumI4OutMax=[]  SumDOutMin=[]  SumDOutMax=[]  DifferentiatorOutMin=[]  DifferentiatorOutMax=[]  FilterDiffOutCoefMin=[]  FilterDiffOutCoefMax=[]  ReciprocalOutMin=[]  ReciprocalOutMax=[]  SumDenOutMin=[]  SumDenOutMax=[]  SumNumOutMin=[]  SumNumOutMax=[]  DivideOutMin=[]  DivideOutMax=[]  UdiffTsProdOutMin=[]  UdiffTsProdOutMax=[]  NTsProdOutMin=[]  NTsProdOutMax=[]  UintegralTsProdOutMin=[]  UintegralTsProdOutMax=[]  UngainTsProdOutMin=[]  UngainTsProdOutMax=[]  IntegratorContinuousStateAttributes=''  IntegratorStateMustResolveToSignalObject=off  IntegratorRTWStateStorageClass=Auto  FilterContinuousStateAttributes=''  FilterStateMustResolveToSignalObject=off  FilterRTWStateStorageClass=Auto  ParallelPVariant=InternalParameters  IdealPVariant=Disabled  IVariant=InternalParameters  DVariant=Disabled  IntegratorVariant=Discrete  SatVariant=Disabled  AWVariant=Passthrough  PCopyVariant=Disabled  TRVariant=Disabled  FdbkBlocksVariant=Forward  IdealPFdbkVariant=Disabled  SatFdbkVariant=Disabled  DerivativeFilterVariant=Disabled  NVariant=Disabled  NCopyVariant=Disabled_SignalSpec  FilterICVariant=Disabled  IntegratorICVariant=InternalICs  ExternalResetVariant=Disabled  TRSumVariant=Passthrough  SumFdbkVariant=Disabled  SumVariant=Sum_PI  TsampFilterVariant=InternalTs  TsampNgainVariant=Passthrough  TsampIntegralVariant=Passthrough
  Discrete PID Controller1 : simulink/Continuous/PID Controller  Controller=PI  Form=Parallel  TimeDomain=Discrete-time  UseExternalTs=off  SampleTime=Ts_Power  IntegratorMethod=Forward Euler  ControllerParametersSource=internal  P=Kp_ccsc  I=Ki_ccsc  D=0  UseFilter=on  N=100  TunerSelectOption=Transfer Function Based (PID Tuner App)  InitialConditionSource=internal  InitialConditionForIntegrator=0  InitialConditionForFilter=0  DifferentiatorICPrevScaledInput=0  ExternalReset=none  TrackingMode=off  Kt=1  LimitOutput=off  UpperSaturationLimit=inf  LowerSaturationLimit=-inf  LinearizeAsGain=off  AntiWindupMode=none  Kb=1  POutMin=[]  POutMax=[]  IOutMin=[]  IOutMax=[]  DOutMin=[]  DOutMax=[]  NOutMin=[]  NOutMax=[]  SumOutMin=[]  SumOutMax=[]  SaturationOutMin=[]  SaturationOutMax=[]  PParamMin=[]  PParamMax=[]  IParamMin=[]  IParamMax=[]  DParamMin=[]  DParamMax=[]  NParamMin=[]  NParamMax=[]  KbParamMin=[]  KbParamMax=[]  KtParamMin=[]  KtParamMax=[]  KbOutMin=[]  KbOutMax=[]  KtOutMin=[]  KtOutMax=[]  IntegratorOutMin=[]  IntegratorOutMax=[]  FilterOutMin=[]  FilterOutMax=[]  SumI1OutMin=[]  SumI1OutMax=[]  SumI2OutMin=[]  SumI2OutMax=[]  SumI3OutMin=[]  SumI3OutMax=[]  SumI4OutMin=[]  SumI4OutMax=[]  SumDOutMin=[]  SumDOutMax=[]  DifferentiatorOutMin=[]  DifferentiatorOutMax=[]  FilterDiffOutCoefMin=[]  FilterDiffOutCoefMax=[]  ReciprocalOutMin=[]  ReciprocalOutMax=[]  SumDenOutMin=[]  SumDenOutMax=[]  SumNumOutMin=[]  SumNumOutMax=[]  DivideOutMin=[]  DivideOutMax=[]  UdiffTsProdOutMin=[]  UdiffTsProdOutMax=[]  NTsProdOutMin=[]  NTsProdOutMax=[]  UintegralTsProdOutMin=[]  UintegralTsProdOutMax=[]  UngainTsProdOutMin=[]  UngainTsProdOutMax=[]  IntegratorContinuousStateAttributes=''  IntegratorStateMustResolveToSignalObject=off  IntegratorRTWStateStorageClass=Auto  FilterContinuousStateAttributes=''  FilterStateMustResolveToSignalObject=off  FilterRTWStateStorageClass=Auto  ParallelPVariant=InternalParameters  IdealPVariant=Disabled  IVariant=InternalParameters  DVariant=Disabled  IntegratorVariant=Discrete  SatVariant=Disabled  AWVariant=Passthrough  PCopyVariant=Disabled  TRVariant=Disabled  FdbkBlocksVariant=Forward  IdealPFdbkVariant=Disabled  SatFdbkVariant=Disabled  DerivativeFilterVariant=Disabled  NVariant=Disabled  NCopyVariant=Disabled_SignalSpec  FilterICVariant=Disabled  IntegratorICVariant=InternalICs  ExternalResetVariant=Disabled  TRSumVariant=Passthrough  SumFdbkVariant=Disabled  SumVariant=Sum_PI  TsampFilterVariant=InternalTs  TsampNgainVariant=Passthrough  TsampIntegralVariant=Passthrough
  Gain : Gain  Gain=2*L_arm_pu
  Gain1 : Gain  Gain=2*L_arm_pu
  Mux1 : Mux  Inputs=3
  Sum1 : Sum  Inputs=-+|
  Sum78 : Sum  Inputs=|++
  Sum83 : Sum  Inputs=-+|
  Sum85 : Sum  Inputs=|+-
  m_dq2 : Outport  VectorParamsAs1DForOutWhenUnconnected=off
  wires:
  Constant2/1 -> Sum85/1
  Constant4/1 -> Mux1/3
  Sum1/1 -> Mux1/2
  Discrete PID Controller1/1 -> Sum1/2
  Discrete PID Controller/1 -> Sum78/1
  Mux1/1 -> m_dq2/1
  I_arm/1 -> Demux/1
  Gain/1 -> Sum1/1
  Sum78/1 -> Mux1/1
  Sum85/1 -> Discrete PID Controller/1
  Sum83/1 -> Discrete PID Controller1/1
  Constant1/1 -> Sum83/2
  Demux/2 -> Sum83/1, Gain1/1
  Gain1/1 -> Sum78/2
  Demux/1 -> Sum85/2, Gain/1

== system B2B_HVDC_MMC/Dq0 Control11/Subsystem1/DC voltage control - Outer loop ==
  note: Id_ref
  V_dc_meas : Inport
  V_dc_ref : Inport  Port=2
  Enable : Inport  Port=3
  DC_limit : Inport  Port=4
  Constant1 : Constant  Value=0
  Gain2 : Gain  Gain=1/Vdc_nom
  PI regulator with anti-windup Q : Subsystem  DialogController=POWERSYS.PowerSysDialog  mask(Discrete PI Controller){Kp=Kp_DCreg_r, Ki=Ki_DCreg_r, Par_Limits=[DC_lim(1) DC_lim(2)], Init=0, Ts=Ts_Control}
      mask prompts: Kp "Proportional gain (Kp):"; Ki "Integral gain (Ki):"; Par_Limits "Output limits: [ Upper   Lower ]"; Init "Output initial value:"; Ts "Sample time:"
      mask help: This block implements a discrete PI controller.
      mask init:
      | UpperLimit=Par_Limits(1);
      | LowerLimit=Par_Limits(2);
      | power_initmask();
      mask Help: This block is part of a subset of blocks in the Extras library that does not have documentation associated with it, other than the block mask description.
      mask Display: disp('PI');
  Rate Transition1 : RateTransition  OutPortSampleTime=Ts_Control
  Second-Order Filter2 : spsSecondOrderFilterLib/Second-Order Filter  FilterType=Lowpass  Fo=Fn_filter*0.4  Zeta=Zeta_filter*2  Ts=Ts_Control  Initialize=off  Vac_Init="[0,  0,  60]"  Vdc_Init=0  PlotResponse=off  FreqRange=[0, 500, 1]
  Sum2 : Sum  Inputs=|-+
  Switch3 : Switch  Criteria=u2 > Threshold  SaturateOnIntegerOverflow=off  InputSameDT=off
  Unit Delay1 : UnitDelay  SampleTime=Ts_Power  HasFrameUpgradeWarning=on
  Id_ref : Outport  VectorParamsAs1DForOutWhenUnconnected=off
  wires:
  Constant1/1 -> Switch3/3
  Switch3/1 -> Gain2/1
  V_dc_meas/1 -> Second-Order Filter2/1
  Enable/1 -> Switch3/2
  Sum2/1 -> Switch3/1
  Rate Transition1/1 -> Sum2/1
  Gain2/1 -> PI regulator with anti-windup Q/1(Error)
  PI regulator with anti-windup Q/1(Out) -> Id_ref/1
  DC_limit/1 -> PI regulator with anti-windup Q/2(Limit)
  Unit Delay1/1 -> Rate Transition1/1
  Second-Order Filter2/1 -> Unit Delay1/1
  V_dc_ref/1 -> Sum2/2

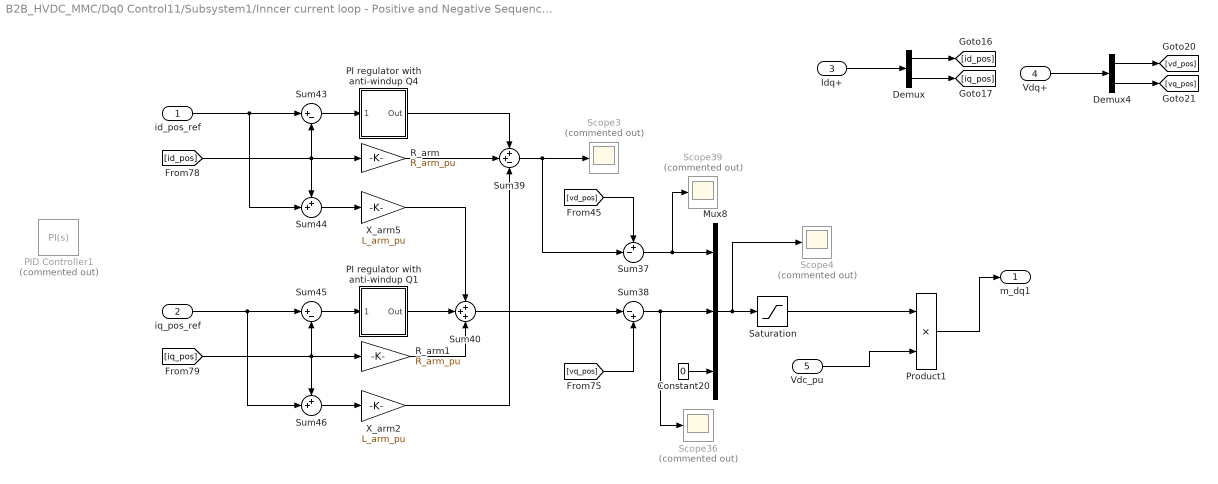
== system B2B_HVDC_MMC/Dq0 Control11/Subsystem1/Inncer current loop - Positive and Negative Sequence Control ==
  id_pos_ref : Inport
  iq_pos_ref : Inport  Port=2
  Idq+ : Inport  Port=3
  Vdq+ : Inport  Port=4
  Vdc_pu : Inport  Port=5
  Constant20 : Constant  Value=0
  Demux : Demux  Outputs=2
  Demux4 : Demux  Outputs=2
  Mux8 : Mux  Inputs=3
  PI regulator with anti-windup Q1 : Subsystem  DialogController=POWERSYS.PowerSysDialog  mask(Discrete PI Controller){Kp=Kp_Ireg_r, Ki=Ki_Ireg_r, Par_Limits=[Ireg_lim_r(1) Ireg_lim_r(2)], Init=0, Ts=Ts_Control}
      mask prompts: Kp "Proportional gain (Kp):"; Ki "Integral gain (Ki):"; Par_Limits "Output limits: [ Upper   Lower ]"; Init "Output initial value:"; Ts "Sample time:"
      mask help: This block implements a discrete PI controller.
      mask init:
      | UpperLimit=Par_Limits(1);
      | LowerLimit=Par_Limits(2);
      | power_initmask();
      mask Help: This block is part of a subset of blocks in the Extras library that does not have documentation associated with it, other than the block mask description.
      mask Display: disp('PI');
  PI regulator with anti-windup Q4 : Subsystem  DialogController=POWERSYS.PowerSysDialog  mask(Discrete PI Controller){Kp=Kp_Ireg_r, Ki=Ki_Ireg_r, Par_Limits=[Ireg_lim_r(1) Ireg_lim_r(2)], Init=0, Ts=Ts_Control}
      mask prompts: Kp "Proportional gain (Kp):"; Ki "Integral gain (Ki):"; Par_Limits "Output limits: [ Upper   Lower ]"; Init "Output initial value:"; Ts "Sample time:"
      mask help: This block implements a discrete PI controller.
      mask init:
      | UpperLimit=Par_Limits(1);
      | LowerLimit=Par_Limits(2);
      | power_initmask();
      mask Help: This block is part of a subset of blocks in the Extras library that does not have documentation associated with it, other than the block mask description.
      mask Display: disp('PI');
  PID Controller1 : simulink/Continuous/PID Controller  Commented=on  Controller=PI  Form=Parallel  TimeDomain=Continuous-time  UseExternalTs=off  SampleTime=-1  IntegratorMethod=Forward Euler  ControllerParametersSource=internal  P=Kp_Ireg_r  I=Ki_Ireg_r  D=0  UseFilter=on  N=100  TunerSelectOption=Transfer Function Based (PID Tuner App)  InitialConditionSource=internal  InitialConditionForIntegrator=0  InitialConditionForFilter=0  DifferentiatorICPrevScaledInput=0  ExternalReset=none  TrackingMode=off  Kt=1  LimitOutput=off  UpperSaturationLimit=inf  LowerSaturationLimit=-inf  LinearizeAsGain=on  AntiWindupMode=none  Kb=1  POutMin=[]  POutMax=[]  IOutMin=[]  IOutMax=[]  DOutMin=[]  DOutMax=[]  NOutMin=[]  NOutMax=[]  SumOutMin=[]  SumOutMax=[]  SaturationOutMin=[]  SaturationOutMax=[]  PParamMin=[]  PParamMax=[]  IParamMin=[]  IParamMax=[]  DParamMin=[]  DParamMax=[]  NParamMin=[]  NParamMax=[]  KbParamMin=[]  KbParamMax=[]  KtParamMin=[]  KtParamMax=[]  KbOutMin=[]  KbOutMax=[]  KtOutMin=[]  KtOutMax=[]  IntegratorOutMin=[]  IntegratorOutMax=[]  FilterOutMin=[]  FilterOutMax=[]  SumI1OutMin=[]  SumI1OutMax=[]  SumI2OutMin=[]  SumI2OutMax=[]  SumI3OutMin=[]  SumI3OutMax=[]  SumI4OutMin=[]  SumI4OutMax=[]  SumDOutMin=[]  SumDOutMax=[]  DifferentiatorOutMin=[]  DifferentiatorOutMax=[]  FilterDiffOutCoefMin=[]  FilterDiffOutCoefMax=[]  ReciprocalOutMin=[]  ReciprocalOutMax=[]  SumDenOutMin=[]  SumDenOutMax=[]  SumNumOutMin=[]  SumNumOutMax=[]  DivideOutMin=[]  DivideOutMax=[]  UdiffTsProdOutMin=[]  UdiffTsProdOutMax=[]  NTsProdOutMin=[]  NTsProdOutMax=[]  UintegralTsProdOutMin=[]  UintegralTsProdOutMax=[]  UngainTsProdOutMin=[]  UngainTsProdOutMax=[]  IntegratorContinuousStateAttributes=''  IntegratorStateMustResolveToSignalObject=off  IntegratorRTWStateStorageClass=Auto  FilterContinuousStateAttributes=''  FilterStateMustResolveToSignalObject=off  FilterRTWStateStorageClass=Auto  ParallelPVariant=InternalParameters  IdealPVariant=Disabled  IVariant=InternalParameters  DVariant=Disabled  IntegratorVariant=Continuous  SatVariant=Disabled  AWVariant=Passthrough  PCopyVariant=Disabled  TRVariant=Disabled  FdbkBlocksVariant=Forward  IdealPFdbkVariant=Disabled  SatFdbkVariant=Disabled  DerivativeFilterVariant=Disabled  NVariant=Disabled  NCopyVariant=Disabled_SignalSpec  FilterICVariant=Disabled  IntegratorICVariant=InternalICs  ExternalResetVariant=Disabled  TRSumVariant=Passthrough  SumFdbkVariant=Disabled  SumVariant=Sum_PI  TsampFilterVariant=InternalTs  TsampNgainVariant=Passthrough  TsampIntegralVariant=Passthrough
  Product1 : Product
  R_arm : Gain  Gain=R_arm_pu
  R_arm1 : Gain  Gain=R_arm_pu
  Saturation : Saturate  UpperLimit=Ireg_lim_r(1)  LowerLimit=Ireg_lim_r(2)
  Scope{3..4,36,39} (4 alike) : Scope  Commented=on
  Sum37 : Sum  Inputs=+-|
  Sum38 : Sum  Inputs=|-+
  Sum39 : Sum  Inputs=++-
  Sum40 : Sum  Inputs=+++
  Sum43 : Sum  Inputs=|+-
  Sum44 : Sum  Inputs=++|
  Sum45 : Sum  Inputs=|+-
  Sum46 : Sum  Inputs=++|
  X_arm2 : Gain  Gain=L_arm_pu
  X_arm5 : Gain  Gain=L_arm_pu
  m_dq1 : Outport  VectorParamsAs1DForOutWhenUnconnected=off
  wires:
  Mux8/1 -> Saturation/1, Scope4/1
  Vdq+/1 -> Demux4/1
  Idq+/1 -> Demux/1
  [id_pos] -> Sum44/1, Sum43/2, R_arm/1
  Demux4/2 -> [vq_pos]
  Demux4/1 -> [vd_pos]
  Vdc_pu/1 -> Product1/2
  Demux/1 -> [id_pos]
  Demux/2 -> [iq_pos]
  Sum45/1 -> PI regulator with anti-windup Q1/1(Error)
  Sum37/1 -> Mux8/1, Scope39/1
  iq_pos_ref/1 -> Sum45/1, Sum46/2
  Sum40/1 -> Sum38/1
  X_arm2/1 -> Sum39/3
  R_arm1/1 -> Sum40/3
  R_arm/1 -> Sum39/2
  Sum44/1 -> X_arm5/1
  Sum43/1 -> PI regulator with anti-windup Q4/1(Error)
  Sum46/1 -> X_arm2/1
  Sum38/1 -> Scope36/1, Mux8/2
  [vd_pos] -> Sum37/1
  [vq_pos] -> Sum38/2
  X_arm5/1 -> Sum40/1
  Sum39/1 -> Sum37/2, Scope3/1
  id_pos_ref/1 -> Sum43/1, Sum44/2
  PI regulator with anti-windup Q1/1(Out) -> Sum40/2
  Constant20/1 -> Mux8/3
  [iq_pos] -> Sum45/2, Sum46/1, R_arm1/1
  PI regulator with anti-windup Q4/1(Out) -> Sum39/1
  Saturation/1 -> Product1/1
  Product1/1 -> m_dq1/1
